simulink model "CAN_SDR_Model"  (R2024a)
settings: Solver=VariableStepAuto  StartTime=0.0  StopTime=10.0  RelTol=1e-3
undefined symbols (not defined in the file): canChannel
libraries: canlib x3, commdigbbndpm3 x2, simulink x2, canmsglib x2, phasedtxrxlib x2, commchan3 x1, dspsigops x1
settings Model: Creator=adcli  LastModifiedBy=adcli
settings RTWCC: GPUComputeCapability=3.5

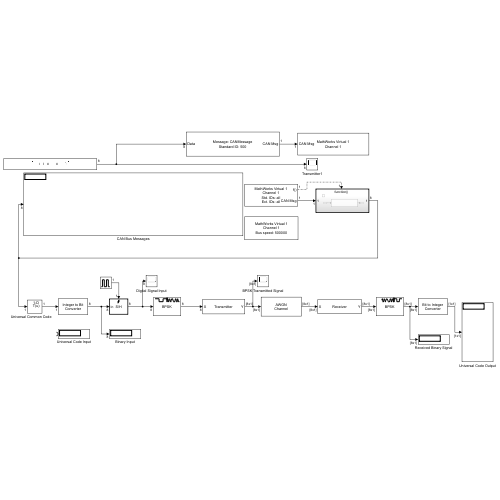
[thumbnail: Simulink's stored preview of the top-level diagram]
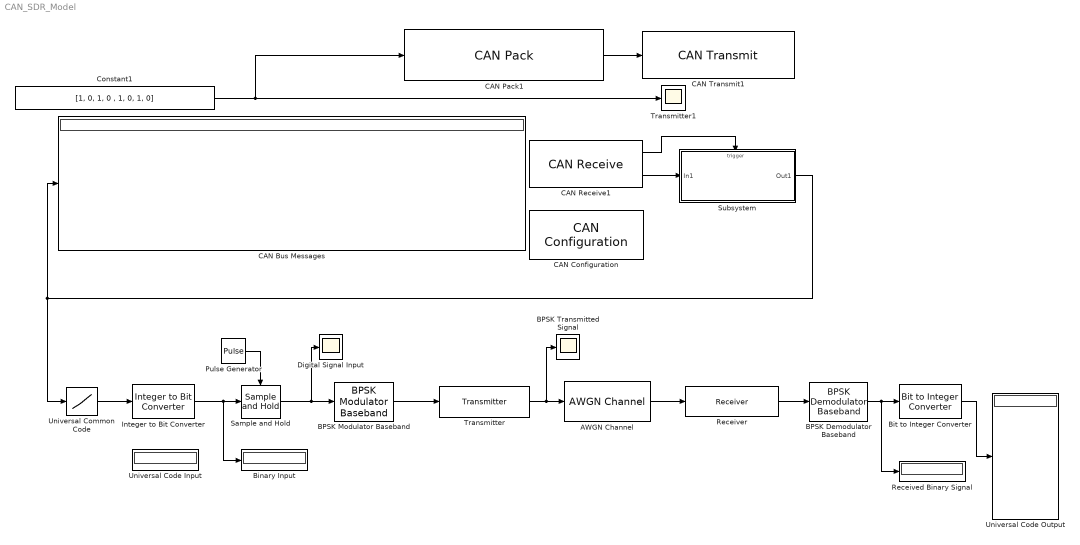
== system CAN_SDR_Model ==
  AWGN Channel : commchan3/AWGN Channel  LegacyMode=off  NoiseMethod="Signal to noise ratio  (SNR)"  noiseMode="Signal to noise ratio  (SNR)"  EbNo=10  EsNo=10  SNR=10  BitsPerSymbol=1  SignalPower=1  SamplesPerSymbol=1  SymbolPeriod=1  VarianceSource=Parameter  Variance=1  RandomStream=Global stream  Seed=67  SimulateUsing=Code generation
  BPSK Demodulator Baseband : commdigbbndpm3/BPSK Demodulator Baseband  DecType=Hard decision  VarSource=Dialog  Variance=1  Ph=0  outDtype=Inherit via internal rule  derotateFactorWordLen=16  derotateFactorDataTypeStr=Inherit: Same word length as input  derotateFactorLastDataTypeStr=Inherit: Same word length as input
  BPSK Modulator Baseband : commdigbbndpm3/BPSK Modulator Baseband  Ph=0  outDtype=double  outWordLen=16  outUDDataType=sfix(16)  outFracLenMode=Best precision  outFracLen=15  outDataTypeStr=double  outLastDataTypeStr=double
  BPSK Transmitted Signal : Scope
  Binary Input : Display
  Bit to Integer Converter : simulink/Logic and Bit Operations/Bit to Integer Converter  nbits=8  bitOrder=MSB first  signedOutputValues=Unsigned  outDtype=Inherit via internal rule  outDtypeSigned=Inherit via internal rule
  CAN Bus Messages : Display
  CAN Configuration : canlib/CAN Configuration  BlockHandle=183.0001  Device=MathWorks Virtual 1 (Channel 1)  DeviceMenu=MathWorks Virtual 1 (Channel 1)  ObjConstructor=canChannel('MathWorks', 'Virtual 1', 1)  BusSpeed=500000  EnableBitParameters=off  AckMode=Normal
  CAN Pack1 : canmsglib/CAN Pack  MsgList=(none)  MsgName=CANMessage  MsgIDType=Standard (11-bit identifier)  MsgIdentifier=500  MsgLength=8  Remote=off  ApplyMinMax=off  BusOutput=off  SignalInfo={'CANSignal','0','64','LE','double','Standard','0','1','0','-1.7e+308','1.7e+308'}
      settings: LibrarySourceBlock=canlib/CAN Pack  DataFormat=raw data
  CAN Receive1 : canlib/CAN Receive  BlockHandle=187.0001  Device=MathWorks Virtual 1 (Channel 1)  DeviceMenu=MathWorks Virtual 1 (Channel 1)  ObjConstructor=canChannel('MathWorks', 'Virtual 1', 1)  EnableStandardIDsFilter=off  StdIDsCombo=Allow all  StandardIDs=0  EnableExtendedIDsFilter=off  ExtIDsCombo=Allow all  ExtendedIDs=0  SampleTime=0.01  MsgsPerTimestep=all  InternalFilterUpdateStatus=on  BusOutput=off
  CAN Transmit1 : canlib/CAN Transmit  BlockHandle=190.0001  Device=MathWorks Virtual 1 (Channel 1)  DeviceMenu=MathWorks Virtual 1 (Channel 1)  ObjConstructor=canChannel('MathWorks', 'Virtual 1', 1)  EnableEventTransmit=off  EnablePeriodicTransmit=off  MessagePeriod=1.000
  Constant1 : Constant  Value=[1, 0, 1, 0 , 1, 0, 1, 0]  OutDataTypeStr=uint8  SampleTime=0.01
  Digital Signal Input : Scope
  Integer to Bit Converter : simulink/Logic and Bit Operations/Integer to Bit Converter  nbits=8  signedInputValues=Unsigned  bitOrder=MSB first  outDtype=Inherit via internal rule
  Pulse Generator : DiscretePulseGenerator  PulseType=Time based  Period=1  PulseWidth=10
  Received Binary Signal : Display
  Receiver : phasedtxrxlib/Receiver  AddInputNoise=off  InputNoiseTemperature=290  NoiseMethod=Noise figure  NoiseFigure=3  NoiseFactor=2  NoiseTemperature=290  ReferenceTemperature=290  SampleRate=1e6  SampleRateFromInputCheckbox=off  SimulateUsing=Interpreted execution  GainMethod=Linear  Gain=20  OIP3=Inf  Table=[ -25, 5, -1; -10, 20, -2; 0, 27, 12; 5, 28, 12 ]  PhaseOffset=0  SeedSource=Auto  Seed=0
  Sample and Hold : dspsigops/Sample and Hold  trig=Rising edge  initCond=0  latchinput=off
  Subsystem : Subsystem
  Transmitter : phasedtxrxlib/Transmitter  PeakPower=5000  GainMethod=Linear  Gain=20  LossFactor=0  OIP3=Inf  Table=[ -25, 5, -1; -10, 20, -2; 0, 27, 12; 5, 28, 12 ]  InUseOutputPort=off  CoherentOnTransmit=on  PhaseNoiseOutputPort=off  SimulateUsing=Interpreted execution  NoiseMethod=None  NoiseFigure=3  NoiseFactor=2  NoiseTemperature=290  ReferenceTemperature=290  SampleRate=1e6  SampleRateFromInputCheckbox=on  PhaseOffset=0  SeedSource=Auto  Seed=0
  Transmitter1 : Scope
  Universal Code Input : Display
  Universal Code Output : Display
  "Universal Common Code       " : Lookup_n-D  NumberOfTableDimensions=1  BreakpointsForDimension1=[0:49]  BreakpointsForDimension1DataTypeStr=uint8  UseOneInputPortForAllInputData=on  Table=[2;0;0;0;10;0;0;0;0;20;0;0;0;0;30;0;0;0;0;40;0;0;0;0;50;0;0;0;0;60;0;0;0;0;70;0;0;0;0;80;0;0;0;0;90;0;0;0;0;100]  TableDataTypeStr=uint8  InterpMethod=Flat  InternalRulePriority=Speed  OutDataTypeStr=double  RndMeth=Simplest  InputSameDT=off
  wires:
  BPSK Demodulator Baseband/1 -> Received Binary Signal/1, Bit to Integer Converter/1
  AWGN Channel/1 -> Receiver/1
  Transmitter/1 -> BPSK Transmitted Signal/1, AWGN Channel/1
  Pulse Generator/1 -> Sample and Hold/Trigger
  Sample and Hold/1 -> Digital Signal Input/1, BPSK Modulator Baseband/1
  Receiver/1 -> BPSK Demodulator Baseband/1
  BPSK Modulator Baseband/1 -> Transmitter/1
  CAN Receive1/1 -> Subsystem/Trigger
  CAN Receive1/2 -> Subsystem/1(In1)
  CAN Pack1/1 -> CAN Transmit1/1
  Bit to Integer Converter/1 -> Universal Code Output/1
  Constant1/1 -> Transmitter1/1, CAN Pack1/1
  Integer to Bit Converter/1 -> Binary Input/1, Sample and Hold/1
  "Universal Common Code       "/1 -> Integer to Bit Converter/1
  Subsystem/1(Out1) -> "Universal Common Code       "/1, CAN Bus Messages/1

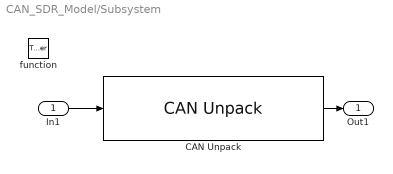
== system CAN_SDR_Model/Subsystem ==
  In1 : Inport
  function : TriggerPort  TriggerType=function-call  VariantControl=(inherit)
  CAN Unpack : canmsglib/CAN Unpack  MsgList=(none)  MsgName=CANMessage  MsgIDType=Standard (11-bit identifier)  MsgIdentifier=500  MsgLength=8  SignalInfo={'CANSignal','0','64','LE','double','Standard','0','1','0','-1.7e+308','1.7e+308'}  IDPort=off  TimestampPort=off  ErrorPort=off  RemotePort=off  LengthPort=off  StatusPort=off  ApplyMinMax=off
      settings: LibrarySourceBlock=canlib/CAN Unpack  DataFormat=raw data
  Out1 : Outport
  wires:
  In1/1 -> CAN Unpack/1
  CAN Unpack/1 -> Out1/1
